simulink model "sim2"  (R2024a)
settings: Solver=FixedStepDiscrete  StartTime=0.0  StopTime=10  FixedStep=0.001  RelTol=1e-3
model workspace (MAT data in the model file):
  Sig = Simulink.Signal
  Sig.DataType = 'auto'
  Sig.Dimensions = -1
  Sig.DimensionsMode = 'auto'
  Sig.Complexity = 'auto'
  Sig.SampleTime = -1
  Sig.SamplingMode = 'auto'
  shift_sw = Simulink.Signal
  shift_sw.DataType = 'auto'
  shift_sw.Dimensions = -1
  shift_sw.DimensionsMode = 'auto'
  shift_sw.Complexity = 'auto'
  shift_sw.SampleTime = -1
  shift_sw.SamplingMode = 'auto'
  speed = Simulink.Signal
  speed.DataType = 'auto'
  speed.Dimensions = -1
  speed.DimensionsMode = 'auto'
  speed.Complexity = 'auto'
  speed.SampleTime = -1
  speed.SamplingMode = 'auto'
  x = Simulink.Signal
  x.DataType = 'auto'
  x.Dimensions = -1
  x.DimensionsMode = 'auto'
  x.Complexity = 'auto'
  x.SampleTime = -1
  x.SamplingMode = 'auto'
  y = Simulink.Signal
  y.DataType = 'auto'
  y.Dimensions = -1
  y.DimensionsMode = 'auto'
  y.Complexity = 'auto'
  y.SampleTime = -1
  y.SamplingMode = 'auto'
undefined symbols (not defined in the file): DD, NN, PP, RR
settings Model: Creator=18283  LastModifiedBy=18283
settings OptimizationCC: DefaultParameterBehavior=Inlined  EnhancedBackFolding=on  PassReuseOutputArgsAs=Individual arguments  ZeroExternalMemoryAtStartup=off  ZeroInternalMemoryAtStartup=off  OptimizeBlockOrder=speed  DifferentSizesBufferReuse=on  OptimizationCustomize=off  EfficientTunableParamExpr=on
settings DebuggingCC: ParameterTunabilityLossMsg=error
settings SFSimCC: MATLABDynamicMemAlloc=off
settings RTWCC: Description=AUTOSAR  SystemTargetFile=autosar.tlc  GenCodeOnly=on  TemplateMakefile=ert_default_tmf  DataTypeReplacement=CDataTypesFixedWidth
settings CodeAppCC: ForceParamTrailComments=on  IgnoreCustomStorageClasses=off  OperatorAnnotations=on  SimulinkDataObjDesc=on  SFDataObjDesc=on  InsertBlockDesc=on
settings STFCustomTargetCC: MultiwordLength=256  ParMdlRefBuildCompliant=on  CompOptLevelCompliant=on  IncludeMdlTerminateFcn=off  CombineOutputUpdateFcns=on  SuppressErrorStatus=on  ERTCustomFileBanners=on  SupportNonFinite=off  SupportComplex=off  SupportContinuousTime=off  SupportNonInlinedSFcns=off  RemoveResetFunc=on  MATLABClassNameForMDSCustomization=Simulink.SoftwareTarget.ERTCustomization  AutosarCompliant=on  GRTInterface=off  LookupTableObjectStructAxisOrder=2,1,3,4,...  LUTObjectStructOrderEvenSpacing=Size,Table,Breakpoints  SystemTargetFile=autosar.tlc
settings ERTTargetCC: TargetLangStandard=C99 (ISO)  ConcurrentExecutionCompliant=off  IncludeMdlTerminateFcn=off  SuppressErrorStatus=on  SupportNonFinite=off  SupportComplex=off  ModelStepFunctionPrototypeControlCompliant=off  CPPClassGenCompliant=off  AutosarCompliant=on  LookupTableObjectStructAxisOrder=2,1,3,4,...  LUTObjectStructOrderEvenSpacing=Size,Table,Breakpoints  InlinedParameterPlacement=NonHierarchical  ERTCustomFileTemplate=example_file_process.tlc  BooleanTrueId=TRUE  BooleanFalseId=FALSE

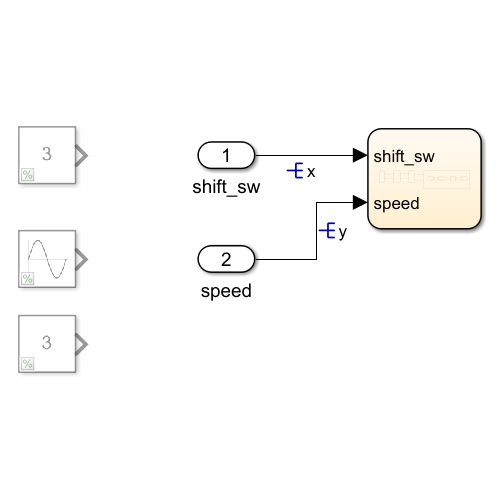
[thumbnail: Simulink's stored preview of the top-level diagram]
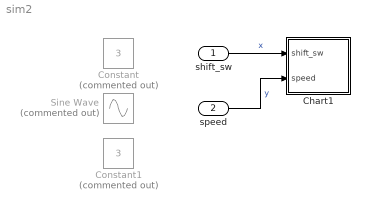
== system sim2 ==
  shift_sw : Inport  OutDataTypeStr=uint8
  speed : Inport  Port=2  OutDataTypeStr=single
  Chart1 : Stateflow chart  TreatAsAtomicUnit=on
  Constant : Constant  Commented=on  Value=3
  Constant1 : Constant  Commented=on  Value=3
  Sine Wave : Sin  Commented=on  Amplitude=100  SampleTime=0
  wires:
  shift_sw/1 -> Chart1/1(shift_sw)  "x"
  speed/1 -> Chart1/2(speed)  "y"

== stateflow chart sim2/Chart1 ==
  state P
  state R
  state N
  state D
    state D1
    state D2
    state D3
    state D4
    (default) -> D1
    D3 -> D4 [order 1] : [speed>60]
    D1 -> D2 : [speed>20]
    D2 -> D3 [order 1] : [speed>40]
    D4 -> D3 : [speed<55]
    D3 -> D2 [order 2] : [speed<35]
    D2 -> D1 [order 2] : [speed<15]
  (default) -> P
  R -> N [order 1] : [shift_sw==NN]
  P -> R : [shift_sw==RR]
  N -> D [order 1] : [shift_sw==DD]
  R -> P [order 2] : [shift_sw==PP]
  N -> R [order 2] : [shift_sw==RR]
  D -> N : [shift_sw==NN]
  data: shift_sw input; speed input; PP parameter; RR parameter; NN parameter; DD parameter
